simulink model "animation"  (Simulink 7.5)
settings: Solver=ode45  StartTime=0.0  StopTime=10000  RelTol=1e-3
undefined symbols (not defined in the file or in its folder): drawMass
libraries: simulink x1
settings Model: Creator=beard  LastModifiedBy=beard
settings OptimizationCC: InitFltsAndDblsToZero=on
settings DebuggingCC: StrictBusMsg=Warning

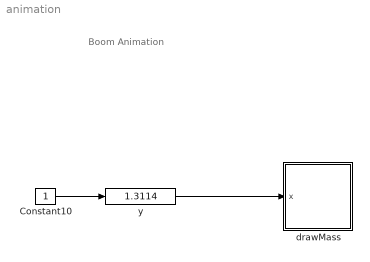
== system animation ==
  note: Boom Animation
  Constant10 : Constant  OutDataType=sfix(16)  OutScaling=2^0
  drawMass : Subsystem
      mask init:
      | % drawing parameters
      | L = 5;
      | w = 1;
      | theta = 45*pi/180;
      mask Display: image(imread('tv.jpg'))
  y : simulink/Math Operations/Slider Gain  SystemSampleTime=-1  low=-10  gain=1.3114  high=10
  wires:
  y/1 -> drawMass/1(x)
  Constant10/1 -> y/1

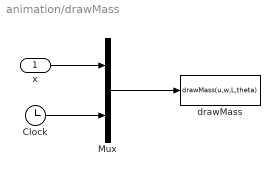
== system animation/drawMass ==
  x : Inport
  Clock : Clock
      settings: Decimation=10
  Mux : Mux  Inputs=2
  drawMass : MATLABFcn  MATLABFcn=drawMass(u,w,L,theta)  OutputDimensions=0  SampleTime=0.1
  wires:
  Mux/1 -> drawMass/1
  x/1 -> Mux/1
  Clock/1 -> Mux/2
